simulink model "Model1"  (R2019b)
settings: Solver=VariableStepAuto  StartTime=0.0  StopTime=10.0  RelTol=1e-3
values from neighbouring files (symbols this model uses):
  g = 9.81    [matlab.mat]
  It = 0.39076347698    [matlab.mat]
  k_am = 3.55200760364    [matlab.mat]
  l1 = 0.000198189411846    [matlab.mat]
  l2 = 0.862122661642    [matlab.mat]
  m = 3.77596397301    [matlab.mat]
libraries: simulink x2
settings Model: OrderedModelArguments=off  Creator=USUARIO  LastModifiedBy=USUARIO

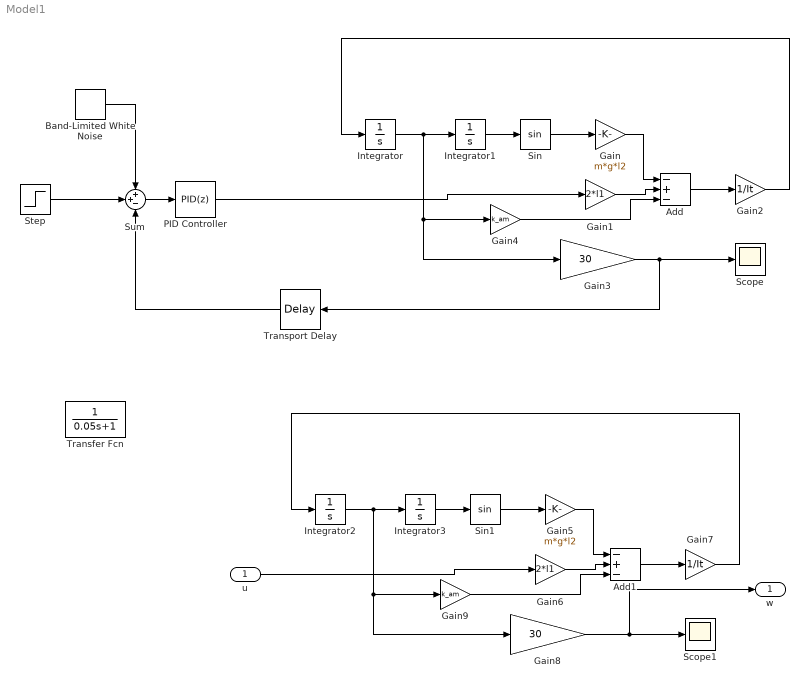
== system Model1 ==
  u : Inport
  Add : Sum  Inputs=-+-
  Add1 : Sum  Inputs=-+-
  Band-Limited White Noise : simulink/Sources/Band-Limited White Noise  Cov=[0.0001]  Ts=0.01  seed=[23341]
  Gain : Gain  Gain=m*g*l2
  Gain1 : Gain  Gain=2*l1
  Gain2 : Gain  Gain=1/It
  Gain3 : Gain  Gain=30
  Gain4 : Gain  Gain=k_am
  Gain5 : Gain  Gain=m*g*l2
  Gain6 : Gain  Gain=2*l1
  Gain7 : Gain  Gain=1/It
  Gain8 : Gain  Gain=30
  Gain9 : Gain  Gain=k_am
  Integrator{,1..3} (4 alike) : Integrator
  PID Controller : simulink/Continuous/PID Controller  Controller=PID  Form=Parallel  TimeDomain=Discrete-time  SampleTime=0.01  IntegratorMethod=Forward Euler  FilterMethod=Forward Euler  ControllerParametersSource=internal  P=107.125309813537  I=511.857911938439  D=4.28232754829949  UseFilter=on  N=99.2432282255825  TunerSelectOption=Transfer Function Based (PID Tuner App)  InitialConditionSource=internal  InitialConditionForIntegrator=0  InitialConditionForFilter=0  DifferentiatorICPrevScaledInput=0  ExternalReset=none  TrackingMode=off  Kt=1  LimitOutput=off  UpperSaturationLimit=inf  LowerSaturationLimit=-inf  LinearizeAsGain=on  AntiWindupMode=none  Kb=1  POutMin=[]  POutMax=[]  IOutMin=[]  IOutMax=[]  DOutMin=[]  DOutMax=[]  NOutMin=[]  NOutMax=[]  SumOutMin=[]  SumOutMax=[]  SaturationOutMin=[]  SaturationOutMax=[]  PParamMin=[]  PParamMax=[]  IParamMin=[]  IParamMax=[]  DParamMin=[]  DParamMax=[]  NParamMin=[]  NParamMax=[]  KbParamMin=[]  KbParamMax=[]  KtParamMin=[]  KtParamMax=[]  KbOutMin=[]  KbOutMax=[]  KtOutMin=[]  KtOutMax=[]  IntegratorOutMin=[]  IntegratorOutMax=[]  FilterOutMin=[]  FilterOutMax=[]  SumI1OutMin=[]  SumI1OutMax=[]  SumI2OutMin=[]  SumI2OutMax=[]  SumI3OutMin=[]  SumI3OutMax=[]  SumI4OutMin=[]  SumI4OutMax=[]  SumDOutMin=[]  SumDOutMax=[]  DifferentiatorOutMin=[]  DifferentiatorOutMax=[]  FilterDiffOutCoefMin=[]  FilterDiffOutCoefMax=[]  ReciprocalOutMin=[]  ReciprocalOutMax=[]  SumDenOutMin=[]  SumDenOutMax=[]  SumNumOutMin=[]  SumNumOutMax=[]  DivideOutMin=[]  DivideOutMax=[]  IntegratorContinuousStateAttributes=''  IntegratorStateMustResolveToSignalObject=off  IntegratorRTWStateStorageClass=Auto  FilterContinuousStateAttributes=''  FilterStateMustResolveToSignalObject=off  FilterRTWStateStorageClass=Auto  ParallelPVariant=InternalParameters  IdealPVariant=Disabled  IVariant=InternalParameters  DVariant=InternalParameters  IntegratorVariant=Discrete  SatVariant=Disabled  AWVariant=Passthrough  PCopyVariant=Disabled  TRVariant=Disabled  FdbkBlocksVariant=Forward  IdealPFdbkVariant=Disabled  SatFdbkVariant=Disabled  DerivativeFilterVariant=ForwardEulerFilter  NVariant=InternalParameters  NCopyVariant=Disabled  FilterICVariant=InternalICsFilter  IntegratorICVariant=InternalICs  ExternalResetVariant=Disabled  TRSumVariant=Passthrough  SumFdbkVariant=Disabled  SumVariant=Sum_PID
  Scope : Scope
  Scope1 : Scope
  Sin : Trigonometry
  Sin1 : Trigonometry
  Step : Step  SampleTime=0
  Sum : Sum  Inputs=++-
  Transfer Fcn : TransferFcn  Denominator=[0.05 1]
  Transport Delay : TransportDelay  DelayTime=0.05
  w : Outport
  wires:
  Integrator/1 -> Gain4/1, Gain3/1, Integrator1/1
  Integrator1/1 -> Sin/1
  Sin/1 -> Gain/1
  Gain/1 -> Add/1
  Gain1/1 -> Add/2
  Add/1 -> Gain2/1
  Gain2/1 -> Integrator/1
  Gain4/1 -> Add/3
  Sum/1 -> PID Controller/1
  Step/1 -> Sum/2
  Gain3/1 -> Transport Delay/1, Scope/1
  Transport Delay/1 -> Sum/3
  PID Controller/1 -> Gain1/1
  Band-Limited White Noise/1 -> Sum/1
  Integrator2/1 -> Gain9/1, Gain8/1, Integrator3/1
  Gain5/1 -> Add1/1
  Gain9/1 -> Add1/3
  Gain8/1 -> w/1, Scope1/1
  Gain7/1 -> Integrator2/1
  Add1/1 -> Gain7/1
  Sin1/1 -> Gain5/1
  Integrator3/1 -> Sin1/1
  Gain6/1 -> Add1/2
  u/1 -> Gain6/1
